simulink model "Mli_com"  (Simulink 8.7)
settings: Solver=FixedStepAuto  StartTime=0.0  StopTime=1  FixedStep=1e-6  RelTol=1e-3
InitFcn:
  | E=220;
libraries: powerlib x14
settings Model: Creator=SINA  LastModifiedBy=SINA
settings DataIOCC: LimitDataPoints=off  SaveFormat=Dataset
settings DebuggingCC: UnderspecifiedInitializationDetection=Simplified  MergeDetectMultiDrivingBlocksExec=error
settings HardwareCC: ProdBitPerPointer=64  ProdLargestAtomicFloat=Float  ProdIntDivRoundTo=Zero  ProdEndianess=LittleEndian  ProdWordSize=64  ProdHWDeviceType=Intel->x86-64 (Windows64)
settings ModelReferenceCC: PropagateSignalLabelsOutOfModel=on
settings ConfigComp: CovModelRefEnable=off

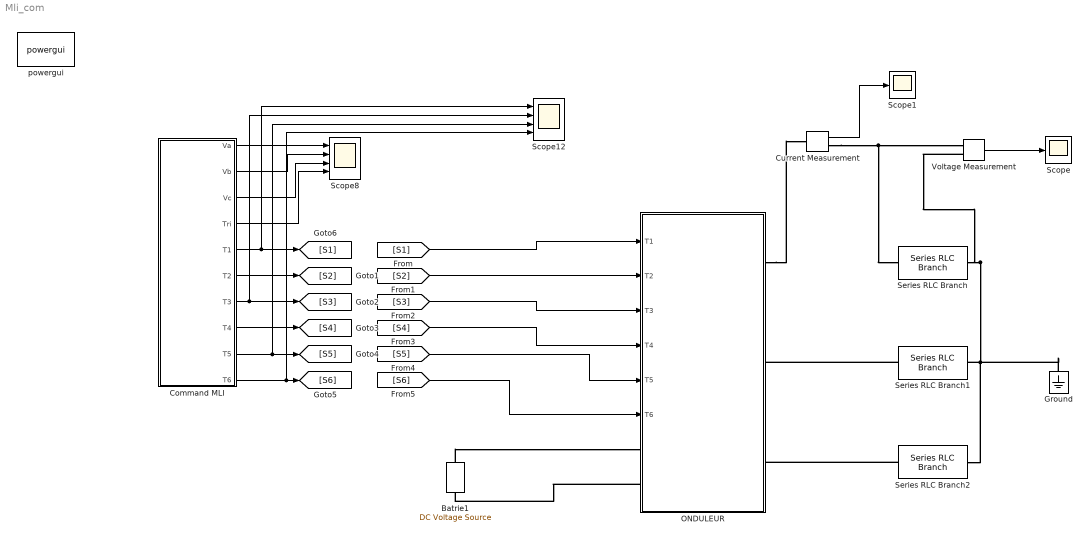
== system Mli_com ==
  Batrie1 : powerlib/Electrical Sources/DC Voltage Source  Amplitude=E  Measurements=Voltage
  Command MLI : Subsystem
  Current Measurement : powerlib/Measurements/Current Measurement  PhasorSimulation=off  OutputType=Complex  PSBequivalent=0
  Ground : powerlib/Elements/Ground  LConnTagsString=a
  ONDULEUR : Subsystem
  Scope : Scope
  Scope1 : Scope
  Scope12 : Scope  NumInputPorts=4
  Scope8 : Scope  NumInputPorts=4
  Series RLC Branch : powerlib/Elements/Series RLC Branch  LConnTagsString=__new0  RConnTagsString=__new0  BranchType=R  Resistance=0.1  Inductance=1e-3  SetiL0=off  InitialCurrent=0  Capacitance=1e-6  Setx0=off  InitialVoltage=0  Measurements=None
  Series RLC Branch1 : powerlib/Elements/Series RLC Branch  LConnTagsString=__new0  RConnTagsString=__new0  BranchType=R  Resistance=0.1  Inductance=1e-3  SetiL0=off  InitialCurrent=0  Capacitance=1e-6  Setx0=off  InitialVoltage=0  Measurements=None
  Series RLC Branch2 : powerlib/Elements/Series RLC Branch  LConnTagsString=__new0  RConnTagsString=__new0  BranchType=R  Resistance=0.1  Inductance=1e-3  SetiL0=off  InitialCurrent=0  Capacitance=1e-6  Setx0=off  InitialVoltage=0  Measurements=None
  Voltage Measurement : powerlib/Measurements/Voltage Measurement  PhasorSimulation=off  OutputType=Complex  PSBequivalent=0
  powergui : powerlib/powergui  Priority=1  SimulationMode=Discrete  SolverType=Tustin/Backward Euler (TBE)  SampleTime=1e-6  frequency=60  SPID=off  DisableSnubberDevices=off  DisableRonSwitches=off  DisableVfSwitches=off  SwTol=0  DisplayEquations=off  Interpol=off  ExternalGateDelay=off  methode=off  Ts=0  FunctionMessages=off  echomessages=off  HookPort=off  EnableUseOfTLC=off  x0status=blocks  frequencyindice=0  Pbase=100e6  ErrMax=1e-4  Iterations=50  UnitsV=kV  UnitsW=MW  buscounter=0  RestoreLinks=warning  ResistiveCurrentMeasurement=off  Frange=[0:2:500]  Ylog=off  Xlog=on  ShowGrid=off  save=off  variable=ZData  structure=0  ZoomFFT=on  StartTime=0.0  cycles=1  DisplayStyle=1  fundamental=60  FreqAxis=off  MaxFrequency=1000  frequencyindicesteady=1  RmsSteady=1  display=off
  wires:
  Command MLI/1(Va) -> Scope8/1
  Command MLI/3(Vc) -> Scope8/3
  Command MLI/4(Tri) -> Scope8/4
  Command MLI/2(Vb) -> Scope8/2
  [S1] -> ONDULEUR/1("T1 ")
  [S3] -> ONDULEUR/3("T3  ")
  [S5] -> ONDULEUR/5("T5 ")
  [S2] -> ONDULEUR/2("T2 ")
  [S4] -> ONDULEUR/4("T4 ")
  [S6] -> ONDULEUR/6("T6 ")
  Command MLI/10(T6) -> Scope12/4, [S6]
  Command MLI/9(T5) -> [S5], Scope12/3
  Command MLI/8(T4) -> [S4]
  Command MLI/7(T3) -> [S3], Scope12/2
  Command MLI/6(T2) -> [S2]
  Command MLI/5(T1) -> [S1], Scope12/1
  Voltage Measurement/1 -> Scope/1
  Current Measurement/1 -> Scope1/1
  connections:
  ONDULEUR/LConn2 -- Batrie1/LConn1
  Batrie1/RConn1 -- ONDULEUR/LConn1
  Series RLC Branch2/LConn1 -- ONDULEUR/RConn3
  Series RLC Branch1/LConn1 -- ONDULEUR/RConn2
  Current Measurement/RConn1 -- Series RLC Branch/LConn1 -- Voltage Measurement/LConn1
  Series RLC Branch/RConn1 -- Voltage Measurement/LConn2 -- Ground/LConn1 -- Series RLC Branch2/RConn1 -- Series RLC Branch1/RConn1
  ONDULEUR/RConn1 -- Current Measurement/LConn1

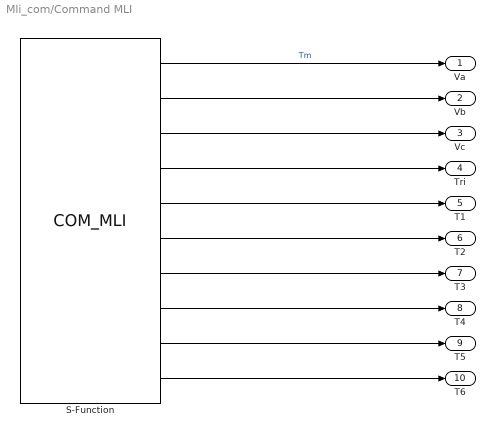
== system Mli_com/Command MLI ==
  S-Function : S-Function  FunctionName=COM_MLI  SFunctionDeploymentMode=off  EnableBusSupport=off
  Va : Outport
  Vb : Outport  Port=2
  Vc : Outport  Port=3
  Tri : Outport  Port=4
  T1 : Outport  Port=5
  T2 : Outport  Port=6
  T3 : Outport  Port=7
  T4 : Outport  Port=8
  T5 : Outport  Port=9
  T6 : Outport  Port=10
  wires:
  S-Function/3 -> Vc/1
  S-Function/2 -> Vb/1
  S-Function/1 -> Va/1  "Tm"
  S-Function/5 -> T1/1
  S-Function/10 -> T6/1
  S-Function/9 -> T5/1
  S-Function/8 -> T4/1
  S-Function/7 -> T3/1
  S-Function/6 -> T2/1
  S-Function/4 -> Tri/1

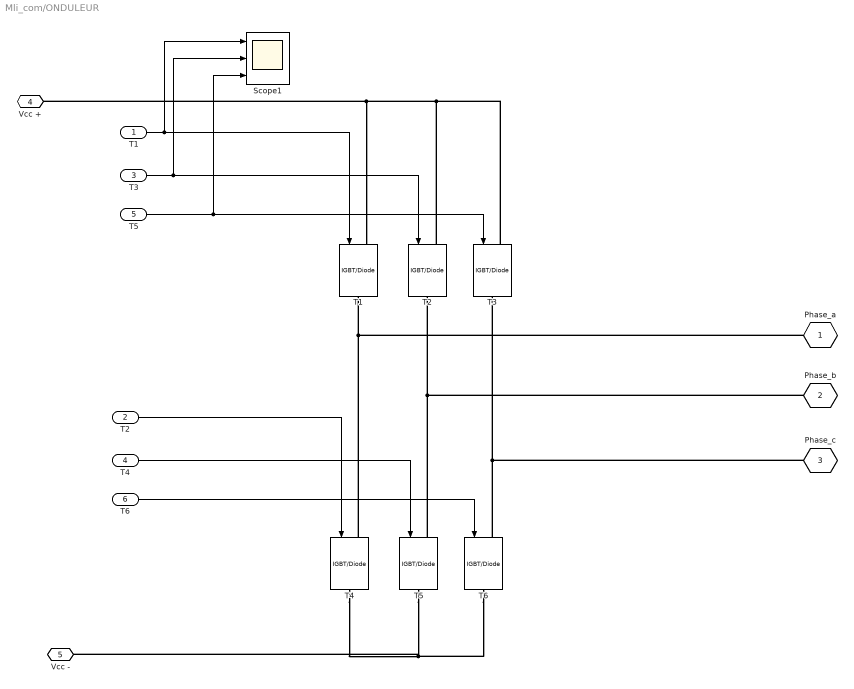
== system Mli_com/ONDULEUR ==
  "T1 " : Inport
  "T2 " : Inport  Port=2
  "T3  " : Inport  Port=3
  "T4 " : Inport  Port=4
  "T5 " : Inport  Port=5
  "T6 " : Inport  Port=6
  Scope1 : Scope  NumInputPorts=3
  T{1..6} (6 alike) : powerlib/Power Electronics/IGBT//Diode  Ron=1e-3  Rs=1e5  Cs=inf  Measurements=off
  Phase_a : PMIOPort  Tag=PMCPort  Port=1  Side=Right
  Phase_b : PMIOPort  Tag=PMCPort  Port=2  Side=Right
  Phase_c : PMIOPort  Tag=PMCPort  Port=3  Side=Right
  Vcc + : PMIOPort  Port=4  Side=Left
  Vcc - : PMIOPort  Port=5  Side=Left
  wires:
  "T1 "/1 -> Scope1/1, T1/1
  "T3  "/1 -> Scope1/2, T2/1
  "T5 "/1 -> Scope1/3, T3/1
  "T2 "/1 -> T4/1
  "T4 "/1 -> T5/1
  "T6 "/1 -> T6/1
  connections:
  T2/LConn1 -- T3/LConn1 -- Vcc +/RConn1 -- T1/LConn1
  T5/RConn1 -- T4/RConn1 -- Vcc -/RConn1 -- T6/RConn1
  T4/LConn1 -- Phase_a/RConn1 -- T1/RConn1
  T5/LConn1 -- Phase_b/RConn1 -- T2/RConn1
  T6/LConn1 -- T3/RConn1 -- Phase_c/RConn1
